simulink model "RoboBoatVU_2014_Eros"  (R2014a)
settings: Solver=FixedStepDiscrete  StartTime=0.0  StopTime=inf  FixedStep=.1  RelTol=1e-3
undefined symbols (not defined in the file): Com1, Com2, Com3, Com4, DiscIntNeverNeededParam, RGB24, standard
libraries: visiontextngfix x68, simulink x53, xpcseriallib x15, dspmtrx3 x14, slrtlib x3, speedgoatlib_IO102 x3, visionstatistics x2, dspstat3 x2, dspindex x2, xpcvideousblib x2, xpcvideoutillib x2, speedgoatlib x1
(part 7 of 7)

== matlab function RoboBoatVU_2014_Eros/Main FSM/Obstacle Navigation/GPS: Bee Line/Orient/Desired Heading ==
  data: DesiredGPS input; DesiredHeading output; GPSLat input; GPSLong input
function DesiredHeading = Orient(DesiredGPS, GPSLat, GPSLong)

%Written by Anderson Lebbad on July 22, 2013
%Last Edited: Edward Zhu on July 5, 2014

% Edit:
% Changed calculation to use positive lat and negative long

%Orients the boat towards a target GPS point before approaching it.
%This is done to keep the approach angle minimal, so the approach
%algorithm does not circle the target and never reach it.

%Parse input GPS and convert angles to radians
CurLat = (floor(GPSLat/100)+mod(GPSLat,100)/60)*pi/180;
CurLong = (ceil(GPSLong/100)-mod(-GPSLong,100)/60)*pi/180;
DesLat = (floor(DesiredGPS(1)/100)+mod(DesiredGPS(1),100)/60)*pi/180;
DesLong = (ceil(DesiredGPS(2)/100)-mod(-DesiredGPS(2),100)/60)*pi/180;

%Difference between longs
DiffLong = DesLong - CurLong;

%Calculate initial bearing - formula documented here: 
%   http://www.movable-type.co.uk/scripts/latlong.html
y = sin(DiffLong)*cos(DesLat);
x = cos(CurLat)*sin(DesLat)-sin(CurLat)*cos(DesLat)*cos(DiffLong);
DesiredHeading = mod(atan2(y, x)*180/pi + 360, 360);

== matlab function RoboBoatVU_2014_Eros/Main FSM/Obstacle Navigation1/Enter Gate/Gate 1 (Red & White)/MATLAB Function ==
  data: Prob input; RPM output; ColorID input; Dist input; Ang input; CurrentHeading input; GPSLat input; GPSLong input; Timer input; DesiredHeading output; gateGPS output
function [RPM,DesiredHeading,gateGPS] = navigation(Prob,ColorID,Dist,Ang,CurrentHeading,GPSLat,GPSLong,Timer)

% Function performs one buoy navigation through the start speed gates. If
% no buoys are found by the LIDAR/Vision assembly then an incremented
% turning algorithm is executed to turn by 10 degrees per increment up to 
% 90 degrees either way of the inital heading

% Written by Edward Zhu

persistent LockHeading TimeLastFound Counter Turn TurnInc gateLat gateLong

if isempty(LockHeading) && isempty(TimeLastFound) && isempty(Counter) && isempty(Turn) && isempty(TurnInc)
    LockHeading = CurrentHeading;
    TimeLastFound = 0;
    Counter = 0;
    TurnInc = 30;
    Turn = TurnInc;
    gateLat = 0;
    gateLong = 0;
end

Distance = Dist/100;

BoatWidth = 0.75;
Buffer = atan(2*BoatWidth/Distance);

RedOffset = Ang + Buffer;
WhiteOffset = Ang - Buffer;

R = 6378137;

CurLat = (floor(GPSLat/100)+mod(GPSLat,100)/60)*pi/180;
CurLong = (ceil(GPSLong/100)-mod(-GPSLong,100)/60)*pi/180;

gateHeading = (mod(CurrentHeading + Ang, 360))*pi/180;

if ColorID == 1 && Prob > 0.9
    if Ang < 0
        DesiredHeading = mod(CurrentHeading - RedOffset, 360);
    else
        DesiredHeading = mod(CurrentHeading + RedOffset, 360);
    end
    RPM = 4000;
    GateFound = 1;
    TimeLastFound = Timer;
    gateLat =  asin(sin(CurLat)*cos(Distance/R) + cos(CurLat)*sin(Distance/R)*cos(gateHeading))*180/pi;
    gateLong = (CurLong + atan2(sin(gateHeading)*sin(Distance/R)*cos(CurLat),cos(Distance/R)-sin(CurLat)*sin(gateLat)))*180/pi;
elseif ColorID == 2 && Prob > 0.9
    DesiredHeading = mod(LockHeading - Turn, 360);
    RPM = 0;
    GateFound = 1;
    TimeLastFound = Timer;
%     DesiredHeading = mod(CurrentHeading - WhiteOffset, 360);
%     RPM = 4000;
%     GateFound = 1;
%     TimeLastFound = Timer;
%     gateLat =  asin(sin(CurLat)*cos(Distance/R) + cos(CurLat)*sin(Distance/R)*cos(gateHeading))*180/pi;
%     gateLong = (CurLong + atan2(sin(gateHeading)*sin(Distance/R)*cos(CurLat),cos(Distance/R)-sin(CurLat)*sin(gateLat)))*180/pi;
else
    DesiredHeading = CurrentHeading;
    RPM = 0;
    GateFound = 0;
end

gateGPS = [gateLat gateLong];
TimeNoBuoys = Timer - TimeLastFound;

if GateFound == 0 && TimeNoBuoys > 15
    RPM = 0;
    DesiredHeading = mod(LockHeading - Turn, 360);
    HeadingDiff = DesiredHeading - CurrentHeading;
    gateGPS = [gateLat gateLong];
    
    if HeadingDiff > 180
        HeadingDiff = HeadingDiff - 360;
    elseif HeadingDiff < -180
        HeadingDiff = HeadingDiff + 360;
    end
    
    if HeadingDiff < 3
        Counter = Counter + 1;
    else
        Counter = 0;
    end
    
    if Counter >= 15
        Turn = Turn + TurnInc;
        Counter = 0;
        if abs(Turn) > 90
            TurnInc = -TurnInc;
        end
    end
end

== matlab function RoboBoatVU_2014_Eros/Main FSM/Communication/Main Enabler ==
  data: taskSelector output; ObstCommEn output; DockingCommEn output; ObstCommFin input
function [taskSelector,ObstCommEn,DockingCommEn] = taskEnabler(ObstCommFin)
%Written by Anderson Lebbad on July 19, 2013
%Last Edited: Edward Zhu on June 2, 2014
%   Substring search for task was written in
%   Case switches were redundant, combined with first set of if statements

%Changes the value of MainMode and the enablers for the tasks within the 
%Main FSM.

% Initialize enable signals
DockingCommEn = 0;
ObstCommEn = 0;

% Set enable signals based on state completion

if ObstCommFin == 0
    ObstCommEn = 1;
    taskSelector = 1;
else
    DockingCommEn = 1;
    taskSelector = 2;
end

== matlab function RoboBoatVU_2014_Eros/Main FSM/Color Sequence Detection/Report/MATLAB Function ==
  data: requestNumOut output; CP input; requestNumIn input; Finished output
function [requestNumOut, Finished] = requestSender(CP, requestNumIn)

if CP < 1
    requestNumOut = requestNumIn;
    Finished = 0;
else
    requestNumOut = 0;
    Finished = 1;
end

== matlab function RoboBoatVU_2014_Eros/Main FSM/Obstacle Navigation1/GPS: Center/GPS Enabler ==
  data: Finished input; GPSMode output; OrientEnable output; ApproachEnable output
function [GPSMode, OrientEnable, ApproachEnable] =...
    GPSEnable(Finished)

%Written by Anderson Lebbad on July 22, 2013
%Last Edited: July 27, 2013
%   Removed Termination Block

%This function enables GPS tasks. First the boat orients towards the
%target, then it approaches it.


%Parse Finished signal
OrientFinished = Finished(1);


%Initialize Enablers
OrientEnable = 0;
ApproachEnable = 0;


%Switches the enable signal based on which task is flagged as done.
if OrientFinished == 0
    OrientEnable = 1;
    GPSMode = 1;
else
    ApproachEnable = 1;
    GPSMode = 2;
end

== matlab function RoboBoatVU_2014_Eros/Main FSM/Obstacle Navigation1/Obstacle Navigation/Dodge/Nav Logic ==
  data: CurrentHeading input; Dist input; Ang input; ObstDist output; RPM output; DesiredHeading output; Timer input; Timeout input; DodgeIncomplete output
 function [ObstDist, RPM, DesiredHeading, DodgeIncomplete] = NavLogic(CurrentHeading,...
    Dist, Ang, Timer, Timeout)

%Written by Anderson Lebbad on August 20, 2013
%Last Edited by:

%Determines the signals for driving through the buoy channel based on the
%bounding box and centroid signals from both the red and green detection
%blocks.

persistent TimeLastFound heldHeading

ObstDist = Dist / 100;

if isempty(TimeLastFound) && isempty(heldHeading)
    TimeLastFound = 0;
    heldHeading = CurrentHeading;
end

if ObstDist > 0 && ObstDist <= 2
    %Buffer for single buoy offset is the angle to twice the boat's width off of the
    %center of the buoy
    BoatWidth = .75;
    Buffer = atan(2 * BoatWidth / ObstDist) * 180 / pi;
    
    if Ang < 0
        ObstOffset = Ang + Buffer;
    else
        ObstOffset = Ang - Buffer;
    end
    
    DesiredHeading = mod(CurrentHeading + ObstOffset, 360);
    RPM = 2800;
    
    TimeLastFound = Timer;
    heldHeading = CurrentHeading;
    
    DodgeIncomplete = 1;
    
else
    DesiredHeading = heldHeading;
    RPM = 2800;
    
    if Timer-TimeLastFound < Timeout
        DodgeIncomplete = 1;
    else
        DodgeIncomplete = 0;
    end

end

== matlab function RoboBoatVU_2014_Eros/Main FSM/Obstacle Navigation1/Obstacle Navigation/MATLAB Function ==
  data: dodgeIncomplete input; dodgeStart input; taskSelector output; dodgeEn output; GPSEn output
function [taskSelector, dodgeEn, GPSEn]  = obstNavEnabler(dodgeIncomplete, dodgeStart)

GPSEn = 0;
dodgeEn = 0;

if  dodgeStart == 1 || dodgeIncomplete == 1
    dodgeEn = 1;
    taskSelector = 1;
else
    GPSEn = 1;
    taskSelector = 2;
end

== matlab function RoboBoatVU_2014_Eros/Main FSM/Main Task Option/Message Composer ==
  data: taskStrInit input; taskStrAdj output
function taskStrAdj = composeMessage(taskStrInit)
%Written by Anderson Lebbad on August 9, 2013
%Last Edited: Edward Zhu on June 2, 2014

%This function adjusts the length of a vector to a set value by filling
%the remaining space with 0's. This is necessary for data store objects
%that have a fixed size for the memory allocation, but a variable length
%input.

%Length of message packet
strLength = 8;

%Size of text in message
taskStrLength = size(taskStrInit,1);

%Pad end of text with zeros
taskStrAdj = [taskStrInit' zeros(1,strLength-taskStrLength)];

== matlab function RoboBoatVU_2014_Eros/Main FSM/Acoustic Location1/GPS: Acoustic Center1/Approach/MATLAB Function ==
  data: PingerAngle input; GPSListenStart output
function GPSListenStart = CheckAngle(PingerAngle)


GPSListenStart = 0;

if PingerAngle ~= 99.99
    GPSListenStart = 1;
end

== matlab function RoboBoatVU_2014_Eros/Main FSM/Acoustic Location1/Acoustic Enabler Block ==
  data: acouLocTask input; GPSWaypointFin input; GPSCenterFin input; ListenFin input; CheckFrontBackFin input; taskSelector output; GPSWaypointEn output; GPSCenterEn output; ListenEn output; CheckFrontBackEn output; GetBuoyDataEn output; ReportBuoyInfoEn output; GetBuoyDataFin input; MovedTooFar input
function [taskSelector,GPSWaypointEn,GPSCenterEn,ListenEn,CheckFrontBackEn,...
    GetBuoyDataEn, ReportBuoyInfoEn] = hydrophoneTestEnabler...
    (acouLocTask, GPSWaypointFin,GPSCenterFin, ListenFin,CheckFrontBackFin,...
    GetBuoyDataFin, MovedTooFar)

%Written by Ed Zhu
%Modified by Michael Benson 7/11/2014 for correct task control

%Changes the value of taskSelector and the enablers for the tasks within the 
%Acoustic Location FSM.

%Initialize enable signals
GPSWaypointEn = 0;
GPSCenterEn = 0;
ListenEn = 0;
CheckFrontBackEn = 0;
GetBuoyDataEn = 0;
ReportBuoyInfoEn = 0;


%Convert data type of task to string
AcouLocStr = char(acouLocTask);


%acouLocTask evaluated to skip certain tasks for testing by flagging them
%as done.

%Check to see if substrings are found by maiking sure the return of strfind
%is not empty
if ~isempty(strfind(AcouLocStr, 'Approach'))
    GPSWaypointFin = 1;
elseif ~isempty(strfind(AcouLocStr, 'Listen'))
    GPSWaypointFin = 1;
    GPSCenterFin = 1;
elseif ~isempty(strfind(AcouLocStr, 'CheckFB'))
    GPSWaypointFin = 1;
    GPSCenterFin = 1;
    ListenFin = 1;
elseif ~isempty(strfind(AcouLocStr, 'GetData'))
    GPSWaypointFin = 1;
    GPSCenterFin = 1;
    ListenFin = 1;
    CheckFrontBackFin = 1;
elseif ~isempty(strfind(AcouLocStr,'Report'))
    GPSWaypointFin = 1;
    GPSCenterFin = 1;
    ListenFin = 1;
    CheckFrontBackFin = 1;
    GetBuoyDataFin = 1;
end

%Switches the enable signal based on which task is flagged as done
if GPSWaypointFin == 0
    GPSWaypointEn = 1;
    taskSelector = 1;
elseif GPSCenterFin == 0
    GPSCenterEn = 1;
    taskSelector = 2;
elseif ListenFin == 0
    ListenEn = 1;
    taskSelector = 3;
elseif CheckFrontBackFin == 0
    CheckFrontBackEn = 1;
    taskSelector = 4;
elseif GetBuoyDataFin == 0
    GetBuoyDataEn = 1;
    taskSelector = 5;
else
    ReportBuoyInfoEn = 1;
    taskSelector = 6;
end

%If, in Listen, the boat moves too far from it's initial position, return
%to the GPS:Center1 task.

if MovedTooFar == 1
    GPSCenterEn = 1;
    ListenEn = 0;
    CheckFrontBackEn = 0;
    taskSelector = 1;
end

== matlab function RoboBoatVU_2014_Eros/Main FSM/Acoustic Location1/GPS:Waypoint/GPS Enabler ==
  data: Finished input; GPSMode output; OrientEn output; ApproachEn output
function [GPSMode, OrientEn, ApproachEn] = GPSEnable(Finished)

%Written by Anderson Lebbad on July 22, 2013
%Last Edited: July 27, 2013
%   Removed Termination Block

%This function enables GPS tasks. First the boat orients towards the
%target, then it approaches it.


%Parse Finished signal
OrientFinished = Finished(1);


%Initialize Enablers
OrientEn = 0;
ApproachEn = 0;


%Switches the enable signal based on which task is flagged as done.
if OrientFinished == 0
    OrientEn = 1;
    GPSMode = 1;
else
    ApproachEn = 1;
    GPSMode = 2;
end

== matlab function RoboBoatVU_2014_Eros/Main FSM/Acoustic Location1/Listen/Listen ==
  data: Timer input; Angle input; Heading input; CurrentLat input; CurrentLong input; Finished output; MovedTooFar output; DesiredHeading output
function [Finished, MovedTooFar, DesiredHeading] = Listen(...
    Timer, Angle, Heading, CurrentLat, CurrentLong)

%%  Written by Michael benson, 7/11/2014
%
%   This code holds heading, and listens to the Arudino Due for pinger
%   angle information.  If the angle is found to be consistent for a few
%   samples, the program terminates.  If the boat moves too far from its
%   initial GPS position, the program terminates and MovedTooFar is set
%   high, which will cause the entire task to revert back to the
%   GPS:Center1 task.

Finished = 0;
MovedTooFar = 0;
PingerAngle = 0;

persistent holdHeading initialLat initialLong lastAngle lastPingTime ...
    startChecker

%%  Initialize persistent variables
if isempty(holdHeading) && isempty(initialLat) && isempty(initialLong) ...
        && isempty(lastAngle) && isempty(lastPingTime) && ...
        isempty(startChecker)
    holdHeading = Heading;
    initialLat = CurrentLat;
    initialLong = CurrentLong;
    lastAngle = 180;
    lastPingTime = 0;
    startChecker = 1;
end

%%  Maintain initial heading
HeadingDiff = abs(holdHeading - Heading);
if HeadingDiff < 4
    DesiredHeading = Heading;
else
    DesiredHeading = holdHeading;
end

%%  Check if boat has moved too far from initial GPS point
DistanceThresh = 3;

initialLatRad = (floor(initialLat/100)+mod(initialLat,100)/60)*pi/180;
initialLongRad = (ceil(initialLong/100)-mod(-initialLong,100)/60)*pi/180;
LatRad = (floor(CurrentLat/100)+mod(CurrentLat,100)/60)*pi/180;
LongRad = (ceil(CurrentLong/100)-mod(-CurrentLong,100)/60)*pi/180;

%Difference between lats and longs
DiffLat = LatRad - initialLatRad;
MidLat = cos((LatRad + initialLatRad)/2);
DiffLong = LongRad - initialLongRad;

%Radius of the earth in meters
R = 6378137;

%Calculating distance using equirectangular approximation since distances
%concerned are very small
a = DiffLong*MidLat;
b = DiffLat;
Distance = R*sqrt(a^2+b^2);


if Distance > DistanceThresh
    MovedTooFar = 1;
end

%%  Register pinger data for first 5 seconds
if Timer < 5 && startChecker == 1 && Angle ~= 99.99
    if Angle ~= lastAngle
        lastPingTime = Timer;
        startChecker = 0;
    end
end


%%  Checks if the angle received from the Due is similar to the previous 
%   angle.  If the difference is within a certain threshold, and the time
%   difference makes sense, the program finishes.
AngleThresh = 10;

TimeDiff = Timer - lastPingTime;
AngleDiff = abs(Angle - lastAngle);

if AngleDiff ~= 0 && TimeDiff > 1.8 && startChecker == 0 && Angle ~= 99.99
    if AngleDiff < AngleThresh && TimeDiff < 8.2
        Finished = 1;
    else
        lastAngle = Angle;
        lastPingTime = Timer;
    end
end
